simulink model "Espaco_Estados_ESC_2DOF_3DOF"  (R2016a)
settings: Solver=VariableStepAuto  StartTime=0.0  StopTime=10  RelTol=1e-3
values from neighbouring files (symbols this model uses):
  A_2 = -E\F    [Espaco_Estados_2DOF_3DOF_Controlador.m]    (also in Parametros_Controller_2_3_DOF.m; Parametros_Controller_2_3_DOF_state_space.m)
  A_3 = -E\F    [Espaco_Estados_2DOF_3DOF_Controlador.m]    (also in Parametros_Controller_2_3_DOF.m; Parametros_Controller_2_3_DOF_state_space.m)
  Bu_2 = E\G    [Espaco_Estados_2DOF_3DOF_Controlador.m]    (also in Parametros_Controller_2_3_DOF.m; Parametros_Controller_2_3_DOF_state_space.m)
  Bu_3 = E\G    [Espaco_Estados_2DOF_3DOF_Controlador.m]    (also in Parametros_Controller_2_3_DOF.m; Parametros_Controller_2_3_DOF_state_space.m)
  Bw_2 = E\H    [Espaco_Estados_2DOF_3DOF_Controlador.m]    (also in Parametros_Controller_2_3_DOF.m; Parametros_Controller_2_3_DOF_state_space.m)
  Bw_3 = E\H    [Espaco_Estados_2DOF_3DOF_Controlador.m]    (also in Parametros_Controller_2_3_DOF.m; Parametros_Controller_2_3_DOF_state_space.m)
  g = 9.81    [Espaco_Estados_2DOF_3DOF_Controlador.m]    (also in Parametros_Controller_2_3_DOF.m; Parametros_Controller_2_3_DOF_state_space.m)
  G1 = u0/(L+Kus*u0^2)    (= 8.7489063867)    [Espaco_Estados_2DOF_3DOF_Controlador.m]    (also in Parametros_Controller_2_3_DOF.m; Parametros_Controller_2_3_DOF_state_space.m)
  K_2 = place(A_lin_2,B_lin_2,polos_2)    [Espaco_Estados_2DOF_3DOF_Controlador.m]
  K_3 = place(A_lin_3,B_lin_3,polos_3)    [Espaco_Estados_2DOF_3DOF_Controlador.m]
  limite_beta = 2.0*(pi/180)    (= 0.0349065850399)    [Espaco_Estados_2DOF_3DOF_Controlador.m]    (also in Parametros_Controller_2_3_DOF.m; Parametros_Controller_2_3_DOF_state_space.m)
  limite_high = (1+delta)*limite_beta    (= 0.0418879020479)    [Espaco_Estados_2DOF_3DOF_Controlador.m]    (also in Parametros_Controller_2_3_DOF.m; Parametros_Controller_2_3_DOF_state_space.m)
  limite_low = (1-delta)*limite_beta    (= 0.0279252680319)    [Espaco_Estados_2DOF_3DOF_Controlador.m]    (also in Parametros_Controller_2_3_DOF.m; Parametros_Controller_2_3_DOF_state_space.m)
  limite_yaw = 1.0*(pi/180)    (= 0.0174532925199)    [Espaco_Estados_2DOF_3DOF_Controlador.m]    (also in Parametros_Controller_2_3_DOF.m; Parametros_Controller_2_3_DOF_state_space.m)
  mu = 0.6    [Espaco_Estados_2DOF_3DOF_Controlador.m]    (also in Parametros_Controller_2_3_DOF.m; Parametros_Controller_2_3_DOF_state_space.m)
  u0 = 80/3.6    (= 22.2222222222)    [Espaco_Estados_2DOF_3DOF_Controlador.m]    (also in Parametros_Controller_2_3_DOF.m; Parametros_Controller_2_3_DOF_state_space.m)
settings Model: Creator=andre  LastModifiedBy=andre
settings DataIOCC: SaveFormat=Array

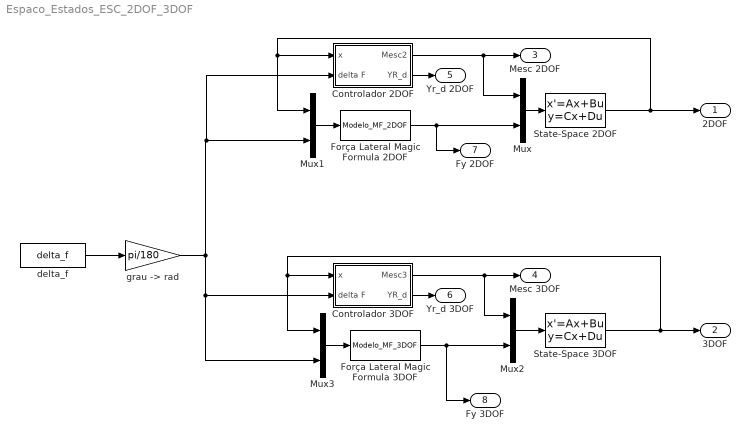
== system Espaco_Estados_ESC_2DOF_3DOF ==
  Controlador 2DOF : Subsystem
  Controlador 3DOF : Subsystem
  Força Lateral Magic Formula 2DOF : MATLABFcn  MATLABFcn=Modelo_MF_2DOF  OutputDimensions=2
  Força Lateral Magic Formula 3DOF : MATLABFcn  MATLABFcn=Modelo_MF_3DOF  OutputDimensions=2
  Mux{,1..3} (4 alike) : Mux  Inputs=2
  State-Space 2DOF : StateSpace  A=A_2  B=[Bu_2 Bw_2]  C=eye(2)  D=zeros(2,3)  X0=0
  State-Space 3DOF : StateSpace  A=A_3  B=[Bu_3 Bw_3]  C=eye(4)  D=zeros(4,3)  X0=0
  delta_f : FromWorkspace  VariableName=delta_f  SampleTime=0
  "grau -> rad" : Gain  Gain=pi/180
  2DOF : Outport  LockScale=on
  3DOF : Outport  Port=2
  Mesc 2DOF : Outport  Port=3  LockScale=on
  Mesc 3DOF : Outport  Port=4  LockScale=on
  Yr_d 2DOF : Outport  Port=5  LockScale=on
  Yr_d 3DOF : Outport  Port=6  LockScale=on
  Fy 2DOF : Outport  Port=7  LockScale=on
  Fy 3DOF : Outport  Port=8  LockScale=on
  wires:
  Mux/1 -> State-Space 2DOF/1
  Força Lateral Magic Formula 2DOF/1 -> Fy 2DOF/1, Mux/2
  Mux1/1 -> Força Lateral Magic Formula 2DOF/1
  State-Space 2DOF/1 -> 2DOF/1, Mux1/1, Controlador 2DOF/1(x)
  Mux2/1 -> State-Space 3DOF/1
  Força Lateral Magic Formula 3DOF/1 -> Fy 3DOF/1, Mux2/2
  Controlador 3DOF/1(Mesc3) -> Mesc 3DOF/1, Mux2/1
  Mux3/1 -> Força Lateral Magic Formula 3DOF/1
  State-Space 3DOF/1 -> 3DOF/1, Controlador 3DOF/1(x), Mux3/1
  "grau -> rad"/1 -> Controlador 3DOF/2(delta F), Mux3/2, Controlador 2DOF/2(delta F), Mux1/2
  delta_f/1 -> "grau -> rad"/1
  Controlador 2DOF/1(Mesc2) -> Mesc 2DOF/1, Mux/1
  Controlador 2DOF/2(YR_d) -> Yr_d 2DOF/1
  Controlador 3DOF/2(YR_d) -> Yr_d 3DOF/1

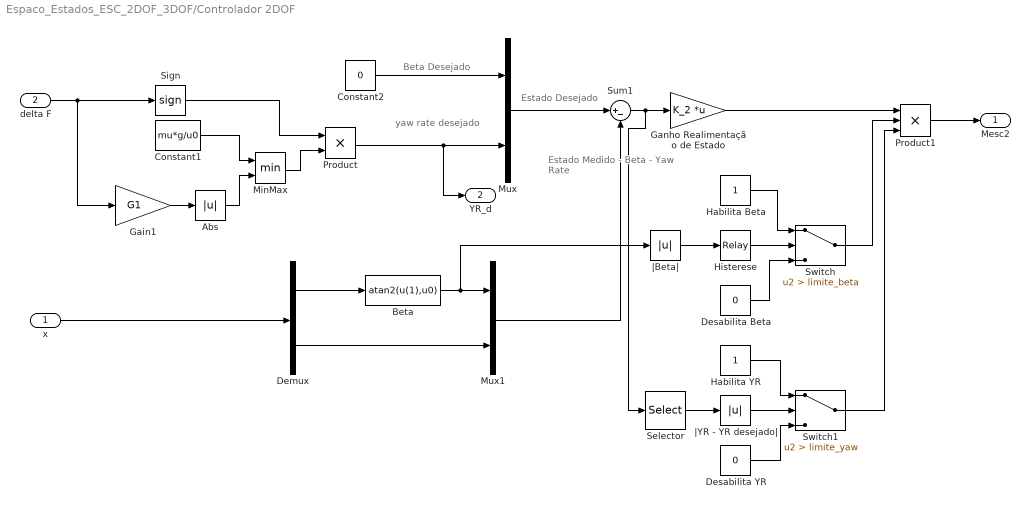
== system Espaco_Estados_ESC_2DOF_3DOF/Controlador 2DOF ==
  note: yaw rate desejado
  note: Beta Desejado
  note: Estado Desejado
  note: Estado Medido
      | - Beta
      | - Yaw Rate
  x : Inport
  delta F : Inport  Port=2
  Abs : Abs
  Beta : Fcn  Expr=atan2(u(1),u0)
  Constant1 : Constant  Value=mu*g/u0
  Constant2 : Constant  Value=0
  Demux : Demux  Outputs=2
  Desabilita Beta : Constant  Value=0
  Desabilita YR : Constant  Value=0
  Gain1 : Gain  Gain=G1
  Ganho Realimentação de Estado : Gain  Gain=K_2  Multiplication=Matrix(K*u)
  Habilita Beta : Constant
  Habilita YR : Constant
  Histerese : Relay  OnSwitchValue=limite_high  OffSwitchValue=limite_low
  MinMax : MinMax  Inputs=2
  Mux : Mux  Inputs=2
  Mux1 : Mux  Inputs=2
  Product : Product
  Product1 : Product  Inputs=3
  Selector : Selector  InputPortWidth=2  IndexOptions=Index vector (dialog)  Indices=[2]  OutputSizes=1
  Sign : Signum
  Sum1 : Sum  Inputs=|+-
  Switch : Switch  Criteria=u2 > Threshold  Threshold=limite_beta
  Switch1 : Switch  Criteria=u2 > Threshold  Threshold=limite_yaw  ZeroCross=off
  |Beta| : Abs
  |YR - YR desejado| : Abs
  Mesc2 : Outport
  YR_d : Outport  Port=2
  wires:
  delta F/1 -> Gain1/1, Sign/1
  Gain1/1 -> Abs/1
  Abs/1 -> MinMax/2
  Constant1/1 -> MinMax/1
  MinMax/1 -> Product/2
  Sign/1 -> Product/1
  Product/1 -> YR_d/1, Mux/2
  Constant2/1 -> Mux/1
  x/1 -> Demux/1
  Demux/2 -> Mux1/2
  Beta/1 -> |Beta|/1, Mux1/1
  Demux/1 -> Beta/1
  Mux1/1 -> Sum1/2
  Sum1/1 -> Selector/1, Ganho Realimentação de Estado/1
  Mux/1 -> Sum1/1
  |Beta|/1 -> Histerese/1
  Histerese/1 -> Switch/2
  Desabilita Beta/1 -> Switch/3
  Desabilita YR/1 -> Switch1/3
  |YR - YR desejado|/1 -> Switch1/2
  Selector/1 -> |YR - YR desejado|/1
  Habilita Beta/1 -> Switch/1
  Habilita YR/1 -> Switch1/1
  Switch1/1 -> Product1/3
  Switch/1 -> Product1/2
  Ganho Realimentação de Estado/1 -> Product1/1
  Product1/1 -> Mesc2/1

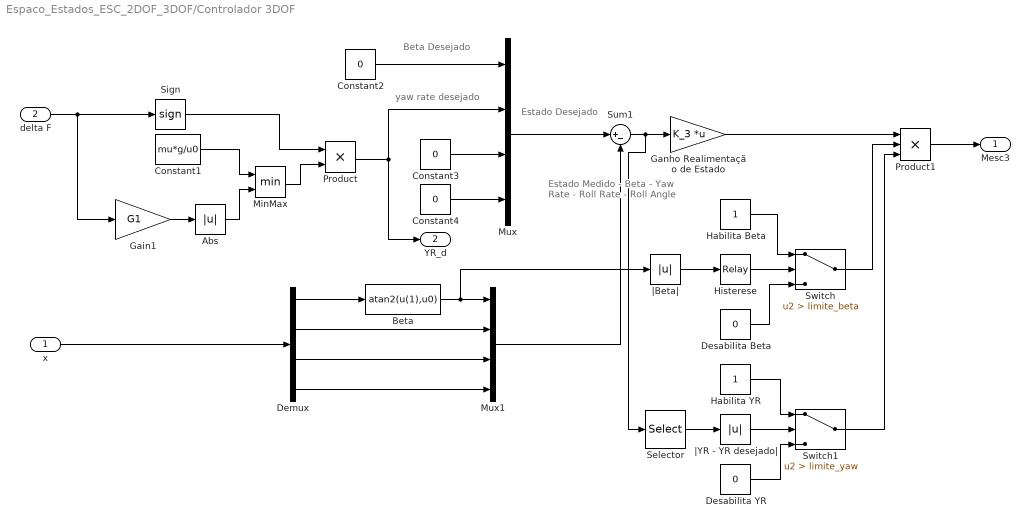
== system Espaco_Estados_ESC_2DOF_3DOF/Controlador 3DOF ==
  note: Estado Medido
      | - Beta
      | - Yaw Rate
      | - Roll Rate
      | - Roll Angle
  note: Estado Desejado
  note: Beta Desejado
  note: yaw rate desejado
  x : Inport
  delta F : Inport  Port=2
  Abs : Abs
  Beta : Fcn  Expr=atan2(u(1),u0)
  Constant1 : Constant  Value=mu*g/u0
  Constant2 : Constant  Value=0
  Constant3 : Constant  Value=0
  Constant4 : Constant  Value=0
  Demux : Demux
  Desabilita Beta : Constant  Value=0
  Desabilita YR : Constant  Value=0
  Gain1 : Gain  Gain=G1
  Ganho Realimentação de Estado : Gain  Gain=K_3  Multiplication=Matrix(K*u)
  Habilita Beta : Constant
  Habilita YR : Constant
  Histerese : Relay  OnSwitchValue=limite_high  OffSwitchValue=limite_low
  MinMax : MinMax  Inputs=2
  Mux : Mux
  Mux1 : Mux
  Product : Product
  Product1 : Product  Inputs=3
  Selector : Selector  InputPortWidth=4  IndexOptions=Index vector (dialog)  Indices=[2]  OutputSizes=1
  Sign : Signum
  Sum1 : Sum  Inputs=|+-
  Switch : Switch  Criteria=u2 > Threshold  Threshold=limite_beta
  Switch1 : Switch  Criteria=u2 > Threshold  Threshold=limite_yaw  ZeroCross=off
  |Beta| : Abs
  |YR - YR desejado| : Abs
  Mesc3 : Outport
  YR_d : Outport  Port=2
  wires:
  Product1/1 -> Mesc3/1
  Ganho Realimentação de Estado/1 -> Product1/1
  Switch/1 -> Product1/2
  Switch1/1 -> Product1/3
  Habilita YR/1 -> Switch1/1
  Habilita Beta/1 -> Switch/1
  Selector/1 -> |YR - YR desejado|/1
  |YR - YR desejado|/1 -> Switch1/2
  Desabilita YR/1 -> Switch1/3
  Desabilita Beta/1 -> Switch/3
  Histerese/1 -> Switch/2
  |Beta|/1 -> Histerese/1
  Mux/1 -> Sum1/1
  Sum1/1 -> Ganho Realimentação de Estado/1, Selector/1
  Mux1/1 -> Sum1/2
  Demux/1 -> Beta/1
  Beta/1 -> |Beta|/1, Mux1/1
  Demux/2 -> Mux1/2
  x/1 -> Demux/1
  Constant2/1 -> Mux/1
  Product/1 -> Mux/2, YR_d/1
  Sign/1 -> Product/1
  MinMax/1 -> Product/2
  Constant1/1 -> MinMax/1
  Abs/1 -> MinMax/2
  Gain1/1 -> Abs/1
  delta F/1 -> Sign/1, Gain1/1
  Constant3/1 -> Mux/3
  Constant4/1 -> Mux/4
  Demux/3 -> Mux1/3
  Demux/4 -> Mux1/4
